simulink model "exp5"  (R2013a)
settings: Solver=ode45  StartTime=0.0  StopTime=10.0  RelTol=1e-3
settings Model: Creator=Karan  LastModifiedBy=Karan

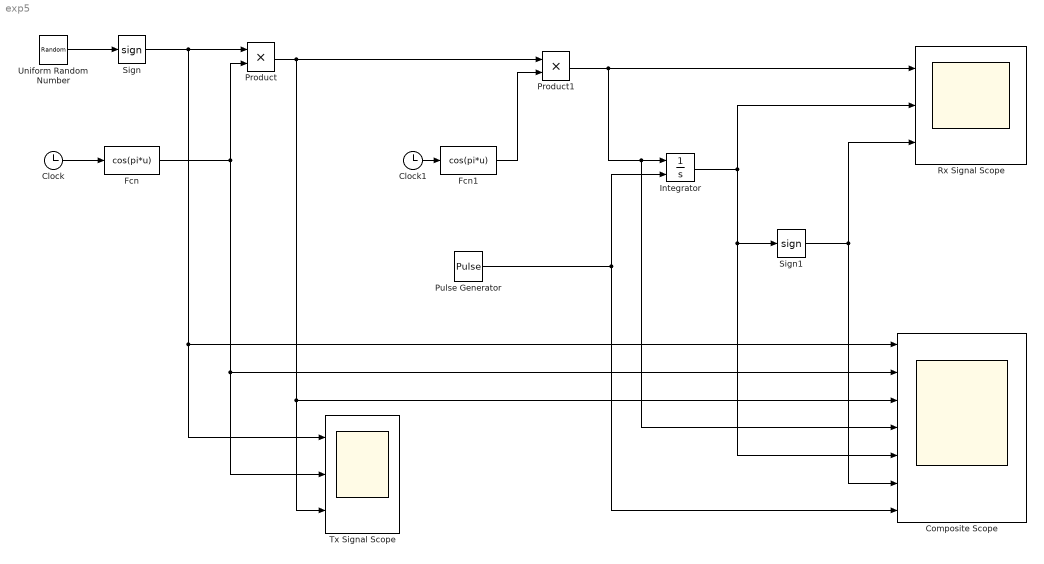
== system exp5 ==
  Clock : Clock
  Clock1 : Clock
  Composite Scope : Scope  NumInputPorts=7
      settings: YMin=-5~-5~-5~-5~-5~-5~-5  YMax=5~5~5~5~5~5~5
  Fcn : Fcn  Expr=cos(pi*u)
  Fcn1 : Fcn  Expr=cos(pi*u)
  Integrator : Integrator  ExternalReset=rising
  Product : Product
  Product1 : Product
  Pulse Generator : DiscretePulseGenerator  PulseType=Time based  Amplitude=5  Period=10  PulseWidth=50
  Rx Signal Scope : Scope  NumInputPorts=3
      settings: YMin=-5~-5~-5  YMax=5~5~5  SaveName=ScopeData2
  Sign : Signum
  Sign1 : Signum
  Tx Signal Scope : Scope  NumInputPorts=3
      settings: YMin=-5~-5~-5  YMax=5~5~5
  Uniform Random Number : UniformRandomNumber  SampleTime=0.1
  wires:
  Uniform Random Number/1 -> Sign/1
  Sign/1 -> Product/1, Tx Signal Scope/1, Composite Scope/1
  Clock/1 -> Fcn/1
  Fcn/1 -> Tx Signal Scope/2, Composite Scope/2, Product/2
  Product/1 -> Tx Signal Scope/3, Composite Scope/3, Product1/1
  Fcn1/1 -> Product1/2
  Clock1/1 -> Fcn1/1
  Product1/1 -> Rx Signal Scope/1, Composite Scope/4, Integrator/1
  Pulse Generator/1 -> Composite Scope/7, Integrator/2
  Integrator/1 -> Composite Scope/5, Sign1/1, Rx Signal Scope/2
  Sign1/1 -> Composite Scope/6, Rx Signal Scope/3
